simulink subsystem "PvtSubSys_LATC"  (R2020b)
settings: Solver=VariableStepAuto  StartTime=0.0  StopTime=10.0  RelTol=1e-3
values from neighbouring files (symbols this model uses):
  P_Global_CharSpd_ms : value not decoded    [PubParsGlobal.sldd]
  P_Global_SteeringAngleRatio : value not decoded    [PubParsGlobal.sldd]
  P_Global_WheelBase_m : value not decoded    [PubParsGlobal.sldd]
  P_LCS_A0_Limit = 0.25    [LATC.sldd]    (also in LCS_v05.sldd)
  P_LCS_A1_Limit = 0.002    [LATC.sldd]    (also in LCS_v05.sldd)
  P_LCS_communicationTest = 1.0    [LATC.sldd]    (also in LCS_v05.sldd)
  P_LCS_Current_Offset_Test_SW = 0.0    [LATC.sldd]
  P_LCS_Current_Offset_Test_Value = 0.0    [LATC.sldd]
  P_LCS_Curvature_bp : value not decoded    [LATC.sldd]
  P_LCS_CycleTime = 0.4 0.4 0.4 0.4 0.4 0.4 0.4 0.4 0.4 0.6 0.6 0.6 0.6 0.6 0.6 0.6 0.4 0.4 0.4 0.4 0.4 0.4 0.4 0.4 0.4 0.6 0.6 0.6 0.6 0.6 0.6 0.6 0.4 0.4 0.4 0.4 0.4 0.4 0.4 0.4 0.4 0.6 0.6 0.6 0.6 0.6 0.6 0.6 0.4 0.4 0.4 0.4 0.4 0.4 0.4 0.4 0.4 0.6 0.6 0.6 0.6 0.6 0.6 0.6 0.4 0.4 0.4 0.4 0.4 0.4 0.4 0.4 0.4 0.6 0.6 0.6 0.6 0.6 0.6 0.6 0.4 0.4 0.4 0.4 0.4 0.4 0.4 0.4 0.4 0.6 0.6 0.6 0.6 0.6 0.6 0.6 0.4 0.4 0.4 0.4    [LATC.sldd]
  P_LCS_ESS_AngleSlope_Limit = 2.9    [LATC.sldd]    (also in LCS_v05.sldd)
  P_LCS_IN_Offset_Test_SW = 0.0    [LATC.sldd]    (also in LCS_v05.sldd)
  P_LCS_IN_Offset_Test_Value = 0.0    [LATC.sldd]    (also in LCS_v05.sldd)
  P_LCS_LATC_CurOffsetVehicleSpdLimitValue_degs = 7.0    [LATC.sldd]
  P_LCS_LATC_Du_Max = 20.0    [LATC.sldd]
  P_LCS_LATC_ELKAngleSlope_ratio : value not decoded    [LATC.sldd]
  P_LCS_LATC_ELKMaxLatAcc_ms2 : value not decoded    [LATC.sldd]
  P_LCS_LATC_ESSAngleSlope_ratio : value not decoded    [LATC.sldd]
  P_LCS_LATC_ESSMaxLatAcc_ms2 : value not decoded    [LATC.sldd]
  P_LCS_LATC_LCAngleSlope_ratio : value not decoded    [LATC.sldd]
  P_LCS_LATC_LCCancleMaxLatAcc_ms2 : value not decoded    [LATC.sldd]
  P_LCS_LATC_LCEcoAngleSlope_ratio : value not decoded    [LATC.sldd]
  P_LCS_LATC_LCEcoMaxLatAcc_ms2 : value not decoded    [LATC.sldd]
  P_LCS_LATC_LCKAngleSlope_ratio : value not decoded    [LATC.sldd]
  P_LCS_LATC_LCKIEAngleSlope_ratio : value not decoded    [LATC.sldd]
  P_LCS_LATC_LCKIEMaxLatAcc_ms2 : value not decoded    [LATC.sldd]
  P_LCS_LATC_LCKMaxLatAcc_ms2 : value not decoded    [LATC.sldd]
  P_LCS_LATC_LCNormalAngleSlope_ratio : value not decoded    [LATC.sldd]
  P_LCS_LATC_LCNormalMaxLatAcc_ms2 : value not decoded    [LATC.sldd]
  P_LCS_LATC_LCSportAngleSlope_ratio : value not decoded    [LATC.sldd]
  P_LCS_LATC_LCSportMaxLatAcc_ms2 : value not decoded    [LATC.sldd]
  P_LCS_LATC_LKAAngleSlope_ratio : value not decoded    [LATC.sldd]
  P_LCS_LATC_LKAMaxLatAcc_ms2 : value not decoded    [LATC.sldd]
  P_LCS_LATC_MatrixQ1_st = 0.8 0.8 1.2 1.4 1.4 1.4 2.0 2.2 2.2 2.2 2.2 2.2 2.2 2.2 2.2 2.2 0.8 0.8 1.2 1.4 1.4 1.4 2.0 2.2 2.2 2.2 2.2 2.2 2.2 2.2 2.2 2.2 0.8 0.8 1.2 1.4 1.4 1.4 2.0 2.2 2.2 2.2 2.2 2.2 2.2 2.2 2.2 2.2 0.8 0.8 1.2 1.4 1.4 1.4 2.0 2.2 2.2 2.2 2.2 2.2 2.2 2.2 2.2 2.2 0.8 0.8 1.2 1.4 1.4 1.4 2.0 2.2 2.2 2.2 2.2 2.2 2.2 2.2 2.2 2.2 0.8 0.8 1.2 1.4 1.4 1.4 2.0 2.2 2.2 2.2 2.2 2.2 2.2 2.2 2.2 2.2 0.8 0.8 1.2 1.4    [LATC.sldd]
  P_LCS_LATC_MatrixQ3_st = 20.0 20.0 20.0 20.0 20.0 15.0 15.0 15.0 15.0 15.0 15.0 15.0 15.0 13.0 13.0 13.0 20.0 20.0 20.0 20.0 20.0 15.0 15.0 15.0 15.0 15.0 15.0 15.0 15.0 13.0 13.0 13.0 20.0 20.0 20.0 20.0 20.0 15.0 15.0 15.0 15.0 15.0 15.0 15.0 15.0 13.0 13.0 13.0 20.0 20.0 20.0 20.0 20.0 15.0 15.0 15.0 15.0 15.0 15.0 15.0 15.0 13.0 13.0 13.0 20.0 20.0 20.0 20.0 20.0 15.0 15.0 15.0 15.0 15.0 15.0 15.0 15.0 13.0 13.0 13.0    [LATC.sldd]
  P_LCS_LATC_MatrixR_st = 10.0 10.0 10.0 10.0 10.0 10.0 10.0 15.0 15.0 15.0 15.0 15.0 15.0 15.0 15.0 15.0 10.0 10.0 10.0 10.0 10.0 10.0 10.0 15.0 15.0 15.0 15.0 15.0 15.0 15.0 15.0 15.0 10.0 10.0 10.0 10.0 10.0 10.0 10.0 15.0 15.0 15.0 15.0 15.0 15.0 15.0 15.0 15.0 10.0 10.0 10.0 10.0 10.0 10.0 10.0 15.0 15.0 15.0 15.0 15.0 15.0 15.0 15.0 15.0 10.0 10.0 10.0 10.0 10.0 10.0 10.0 15.0 15.0 15.0 15.0 15.0 15.0 15.0 15.0 15.0    [LATC.sldd]
  P_LCS_LATC_Max_LatAcc = 4.0    [LATC.sldd]
  P_LCS_LATC_Max_Phi = 15.0    [LATC.sldd]
  P_LCS_LATC_Max_y = 0.5    [LATC.sldd]
  P_LCS_LATC_MPC_SW = 0.0    [LATC.sldd]
  P_LCS_LATC_PreView_SW = 1.0    [LATC.sldd]
  P_LCS_LATC_SoftConstWeight = 1.0    [LATC.sldd]
  P_LCS_LATC_StateActivAngleSlopeLimit_ratio : value not decoded    [LATC.sldd]
  P_LCS_LATC_StateActiveFlg_TabX_st : value not decoded    [LATC.sldd]
  P_LCS_LATC_StateActiveHoldTime_TabY_st : value not decoded    [LATC.sldd]
  P_LCS_LATC_StateHoldTime_st = 250.0    [LATC.sldd]
  P_LCS_LATC_TarAngleFliterWindowSize = 5.0    [LATC.sldd]
  P_LCS_LATC_TarAngleLP_Time = 0.02    [LATC.sldd]
  P_LCS_LATC_U_Max = 90.0    [LATC.sldd]
  P_LCS_LCK_AngleSlope_Limit = 1.4    [LATC.sldd]
  P_LCS_LineVaildSW = 0.0    [LATC.sldd]
  P_LCS_Lookahead_Distance : value not decoded    [LATC.sldd]
  P_LCS_Lookahead_DistanceFac : value not decoded    [LATC.sldd]
  P_LCS_PLAN_CurvePreView_s = 0.3    [LATC.sldd]
  P_LCS_PLAN_CurvePreview_TabX_m : value not decoded    [LATC.sldd]
  P_LCS_PLAN_CurvePreViewFilterTime_s = 0.1    [LATC.sldd]
  P_LCS_PLAN_ELKAyDtLimit_Tab_ms3 = 1.0 1.0 1.0 1.0 1.0 1.0 1.0 1.0 1.0 1.0 1.0 1.0 1.0 1.0 1.0 1.0 1.0 1.0 1.0 1.0 1.0 1.0 1.0 1.0 1.0 1.0 1.0 1.0 1.0 1.0 1.0 1.0 1.0 1.0 1.0 1.0 1.0 1.0 1.0 1.0 1.0 1.0 1.0 1.0 1.0 1.0 1.0 1.0 1.0 1.0 1.0 1.0 1.0 1.0 1.0 1.0 1.0 1.0 1.0 1.0 1.0 1.0 1.0 1.0 1.0 1.0 1.0 1.0 1.0 1.0 1.0 1.0 1.0 1.0 1.0 1.0 1.0 1.0 1.0 1.0 1.0 1.0 1.0 1.0 1.0 1.0 1.0 1.0 1.0 1.0 1.0 1.0 1.0 1.0 1.0 1.0 1.0 1.0 1.0 1.0    [LATC.sldd]
  P_LCS_PLAN_ESSAyDtLimit_Tab_ms3 = 1.0 1.0 1.0 1.0 1.0 1.0 1.0 1.0 1.0 1.0 1.0 1.0 1.0 1.0 1.0 1.0 1.0 1.0 1.0 1.0 1.0 1.0 1.0 1.0 1.0 1.0 1.0 1.0 1.0 1.0 1.0 1.0 1.0 1.0 1.0 1.0 1.0 1.0 1.0 1.0 1.0 1.0 1.0 1.0 1.0 1.0 1.0 1.0 1.0 1.0 1.0 1.0 1.0 1.0 1.0 1.0 1.0 1.0 1.0 1.0 1.0 1.0 1.0 1.0 1.0 1.0 1.0 1.0 1.0 1.0 1.0 1.0 1.0 1.0 1.0 1.0 1.0 1.0 1.0 1.0 1.0 1.0 1.0 1.0 1.0 1.0 1.0 1.0 1.0 1.0 1.0 1.0 1.0 1.0 1.0 1.0 1.0 1.0 1.0 1.0    [LATC.sldd]
  P_LCS_PLAN_LCCancleAyDtLimit_Tab_ms3 = 1.0 1.0 1.0 1.0 1.0 1.0 1.0 1.0 1.0 1.0 1.0 1.0 1.0 1.0 1.0 1.0 1.0 1.0 1.0 1.0 1.0 1.0 1.0 1.0 1.0 1.0 1.0 1.0 1.0 1.0 1.0 1.0 1.0 1.0 1.0 1.0 1.0 1.0 1.0 1.0 1.0 1.0 1.0 1.0 1.0 1.0 1.0 1.0 1.0 1.0 1.0 1.0 1.0 1.0 1.0 1.0 1.0 1.0 1.0 1.0 1.0 1.0 1.0 1.0 1.0 1.0 1.0 1.0 1.0 1.0 1.0 1.0 1.0 1.0 1.0 1.0 1.0 1.0 1.0 1.0 1.0 1.0 1.0 1.0 1.0 1.0 1.0 1.0 1.0 1.0 1.0 1.0 1.0 1.0 1.0 1.0 1.0 1.0 1.0 1.0    [LATC.sldd]
  P_LCS_PLAN_LCEcoAyDtLimit_Tab_ms3 = 1.0 1.0 1.0 1.0 1.0 1.0 1.0 1.0 1.0 1.0 1.0 1.0 1.0 1.0 1.0 1.0 1.0 1.0 1.0 1.0 1.0 1.0 1.0 1.0 1.0 1.0 1.0 1.0 1.0 1.0 1.0 1.0 1.0 1.0 1.0 1.0 1.0 1.0 1.0 1.0 1.0 1.0 1.0 1.0 1.0 1.0 1.0 1.0 1.0 1.0 1.0 1.0 1.0 1.0 1.0 1.0 1.0 1.0 1.0 1.0 1.0 1.0 1.0 1.0 1.0 1.0 1.0 1.0 1.0 1.0 1.0 1.0 1.0 1.0 1.0 1.0 1.0 1.0 1.0 1.0 1.0 1.0 1.0 1.0 1.0 1.0 1.0 1.0 1.0 1.0 1.0 1.0 1.0 1.0 1.0 1.0 1.0 1.0 1.0 1.0    [LATC.sldd]
  P_LCS_PLAN_LCKAyDtLimit_Tab_ms3 = 1.5 1.5 1.5 1.5 1.5 1.5 1.5 1.5 1.5 1.5 1.5 1.5 1.5 1.5 1.5 1.5 1.5 1.5 1.5 1.5 1.5 1.5 1.5 1.5 1.5 1.5 1.5 1.5 1.5 1.5 1.5 1.5 1.5 1.5 1.5 1.5 1.5 1.5 1.5 1.5 1.5 1.5 1.5 1.5 1.5 1.5 1.5 1.5 1.5 1.5 1.5 1.5 1.5 1.5 1.5 1.5 1.5 1.5 1.5 1.5 1.5 1.5 1.5 1.5 1.5 1.5 1.5 1.5 1.5 1.5 1.5 1.5 1.5 1.5 1.5 1.5 1.5 1.5 1.5 1.5 1.5 1.5 1.5 1.5 1.5 1.5 1.5 1.5 1.5 1.5 1.5 1.5 1.5 1.5 1.5 1.5 1.5 1.5 1.5 1.5    [LATC.sldd]
  P_LCS_PLAN_LCKIEAyDtLimit_Tab_ms3 = 1.0 1.0 1.0 1.0 1.0 1.0 1.0 1.0 1.0 1.0 1.0 1.0 1.0 1.0 1.0 1.0 1.0 1.0 1.0 1.0 1.0 1.0 1.0 1.0 1.0 1.0 1.0 1.0 1.0 1.0 1.0 1.0 1.0 1.0 1.0 1.0 1.0 1.0 1.0 1.0 1.0 1.0 1.0 1.0 1.0 1.0 1.0 1.0 1.0 1.0 1.0 1.0 1.0 1.0 1.0 1.0 1.0 1.0 1.0 1.0 1.0 1.0 1.0 1.0 1.0 1.0 1.0 1.0 1.0 1.0 1.0 1.0 1.0 1.0 1.0 1.0 1.0 1.0 1.0 1.0 1.0 1.0 1.0 1.0 1.0 1.0 1.0 1.0 1.0 1.0 1.0 1.0 1.0 1.0 1.0 1.0 1.0 1.0 1.0 1.0    [LATC.sldd]
  P_LCS_PLAN_LCNormalAyDtLimit_Tab_ms3 = 1.0 1.0 1.0 1.0 1.0 1.0 1.0 1.0 1.0 1.0 1.0 1.0 1.0 1.0 1.0 1.0 1.0 1.0 1.0 1.0 1.0 1.0 1.0 1.0 1.0 1.0 1.0 1.0 1.0 1.0 1.0 1.0 1.0 1.0 1.0 1.0 1.0 1.0 1.0 1.0 1.0 1.0 1.0 1.0 1.0 1.0 1.0 1.0 1.0 1.0 1.0 1.0 1.0 1.0 1.0 1.0 1.0 1.0 1.0 1.0 1.0 1.0 1.0 1.0 1.0 1.0 1.0 1.0 1.0 1.0 1.0 1.0 1.0 1.0 1.0 1.0 1.0 1.0 1.0 1.0 1.0 1.0 1.0 1.0 1.0 1.0 1.0 1.0 1.0 1.0 1.0 1.0 1.0 1.0 1.0 1.0 1.0 1.0 1.0 1.0    [LATC.sldd]
  P_LCS_PLAN_LCSportAyDtLimit_Tab_ms3 = 1.0 1.0 1.0 1.0 1.0 1.0 1.0 1.0 1.0 1.0 1.0 1.0 1.0 1.0 1.0 1.0 1.0 1.0 1.0 1.0 1.0 1.0 1.0 1.0 1.0 1.0 1.0 1.0 1.0 1.0 1.0 1.0 1.0 1.0 1.0 1.0 1.0 1.0 1.0 1.0 1.0 1.0 1.0 1.0 1.0 1.0 1.0 1.0 1.0 1.0 1.0 1.0 1.0 1.0 1.0 1.0 1.0 1.0 1.0 1.0 1.0 1.0 1.0 1.0 1.0 1.0 1.0 1.0 1.0 1.0 1.0 1.0 1.0 1.0 1.0 1.0 1.0 1.0 1.0 1.0 1.0 1.0 1.0 1.0 1.0 1.0 1.0 1.0 1.0 1.0 1.0 1.0 1.0 1.0 1.0 1.0 1.0 1.0 1.0 1.0    [LATC.sldd]
  P_LCS_PLAN_LKAAyDtLimit_Tab_ms3 = 1.0 1.0 1.0 1.0 1.0 1.0 1.0 1.0 1.0 1.0 1.0 1.0 1.0 1.0 1.0 1.0 1.0 1.0 1.0 1.0 1.0 1.0 1.0 1.0 1.0 1.0 1.0 1.0 1.0 1.0 1.0 1.0 1.0 1.0 1.0 1.0 1.0 1.0 1.0 1.0 1.0 1.0 1.0 1.0 1.0 1.0 1.0 1.0 1.0 1.0 1.0 1.0 1.0 1.0 1.0 1.0 1.0 1.0 1.0 1.0 1.0 1.0 1.0 1.0 1.0 1.0 1.0 1.0 1.0 1.0 1.0 1.0 1.0 1.0 1.0 1.0 1.0 1.0 1.0 1.0 1.0 1.0 1.0 1.0 1.0 1.0 1.0 1.0 1.0 1.0 1.0 1.0 1.0 1.0 1.0 1.0 1.0 1.0 1.0 1.0    [LATC.sldd]
  P_LCS_PLAN_MinPlanDis_m : value not decoded    [LATC.sldd]
  P_LCS_PLAN_PreCurMinDisFac_ratio : value not decoded    [LATC.sldd]
  P_LCS_PLAN_PreDisCurve_TabX_m : value not decoded    [LATC.sldd]
  P_LCS_PLAN_StateActiv_AyDtLimit_ms3 : value not decoded    [LATC.sldd]
  P_LCS_PLAN_VehicleSpd_TabX_kph : value not decoded    [LATC.sldd]
  P_LCS_PLAN_VehicleSpd_TabY_Kph : value not decoded    [LATC.sldd]
  P_LCS_Trq_Switch = 0.0    [LATC.sldd]    (also in LCS_v05.sldd)
  P_LCS_VehicleSpd_TabX_Kph : value not decoded    [LATC.sldd]
undefined symbols (not defined in the file or in its folder): HWP_AngCmdReqVal, HWP_AngCmdReqValVld, HWP_FuncTrqCmdReqFlag, HWP_ReqCtrlEPS, HWP_ReqCtrlEPSVld, HWP_TrqOvlCmdReqValue, HWP_WorkReq, HWP_WorkReqVld
libraries: simulink x4, dspbuff3 x2
(part 3 of 8)

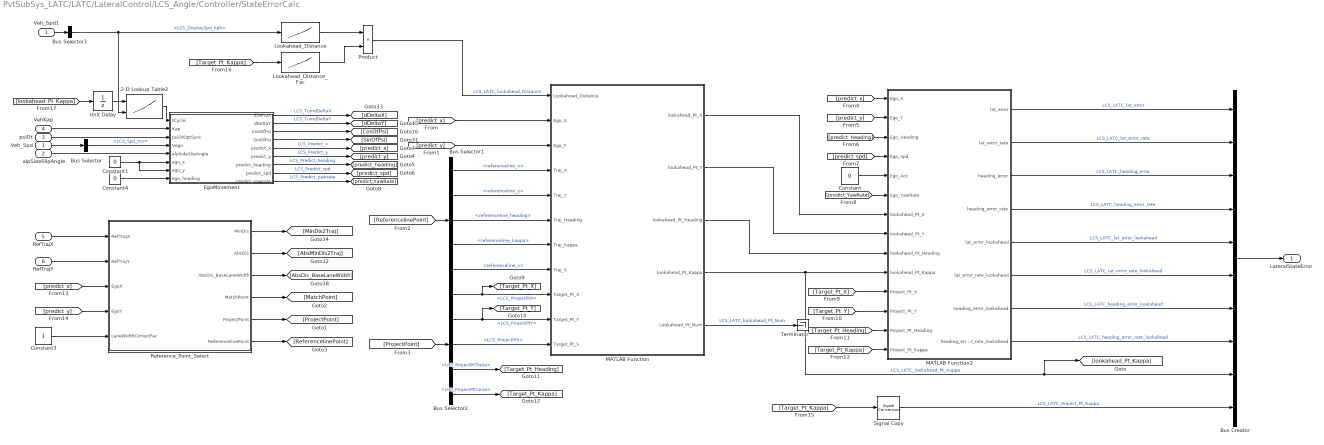
== system PvtSubSys_LATC/LATC/LateralControl/LCS_Angle/Controller/StateErrorCalc ==
  Veh_Spd : Inport
  alpSideSlipAngle : Inport  Port=2
  psiDt : Inport  Port=3
  VehKap : Inport  Port=4
  RefTrajX : Inport  Port=5
  RefTrajY : Inport  Port=6
  2-D Lookup Table2 : Lookup_n-D  BreakpointsForDimension1=P_LCS_Curvature_bp  BreakpointsForDimension2=P_LCS_VehicleSpd_TabX_Kph  Table=P_LCS_CycleTime  InternalRulePriority=Speed  RndMeth=Simplest  InputSameDT=on
      settings: InputPortMap=u0,u1
  Bus Creator : BusCreator  Inputs=10
  Bus Selector : BusSelector  OutputSignals=LCS_Spd_ms
  Bus Selector1 : BusSelector  OutputSignals=referenceline_x,referenceline_y,referenceline_heading,referenceline_kappa,referenceline_s
  Bus Selector2 : BusSelector  OutputSignals=LCS_ProjectPtX,LCS_ProjectPtY,LCS_ProjectPtS,LCS_ProjectPtTheta,LCS_ProjectPtCurve
  Bus Selector3 : BusSelector  OutputSignals=LCS_DisplaySpd_kph
  Constant : Constant  Value=0  OutDataTypeStr=single
  Constant1 : Constant  Value=0  OutDataTypeStr=single
  Constant3 : Constant  OutDataTypeStr=single
  Constant4 : Constant  Value=0  OutDataTypeStr=single
  EgoMovement : MATLAB Function  TreatAsAtomicUnit=on
  Lookahead_Distance : Lookup_n-D  NumberOfTableDimensions=1  BreakpointsForDimension1=P_LCS_VehicleSpd_TabX_Kph  Table=P_LCS_Lookahead_Distance  ExtrapMethod=Clip  UseLastTableValue=on  InternalRulePriority=Speed  RndMeth=Simplest  InputSameDT=on
  Lookahead_Distance_Fac : Lookup_n-D  NumberOfTableDimensions=1  BreakpointsForDimension1=P_LCS_Curvature_bp  Table=P_LCS_Lookahead_DistanceFac  ExtrapMethod=Clip  UseLastTableValue=on  InternalRulePriority=Speed  RndMeth=Simplest  InputSameDT=on
  MATLAB Function : MATLAB Function  TreatAsAtomicUnit=on
  MATLAB Function2 : MATLAB Function  TreatAsAtomicUnit=on
  Product : Product
  Reference_Point_Select : Subsystem
  Signal Copy : SignalConversion  OverrideOpt=off
  Terminator : Terminator
  Unit Delay : UnitDelay  SampleTime=-1  HasFrameUpgradeWarning=on
  Veh_Spd1 : InportShadow
  LateralStateError : Outport
  wires:
  Unit Delay/1 -> 2-D Lookup Table2/1
  Veh_Spd1/1 -> Bus Selector3/1
  [lookahead_Pt_Kappa] -> Unit Delay/1
  2-D Lookup Table2/1 -> EgoMovement/1(tCycle)
  Lookahead_Distance_Fac/1 -> Product/2
  Lookahead_Distance/1 -> Product/1
  [Target_Pt_Kappa] -> Lookahead_Distance_Fac/1
  Bus Selector3/1 -> Lookahead_Distance/1, 2-D Lookup Table2/2  "<LCS_DisplaySpd_kph>"
  [Target_Pt_Kappa] -> Signal Copy/1
  Constant/1 -> MATLAB Function2/5(Ego_Acc)
  MATLAB Function/2(lookahead_Pt_Y) -> MATLAB Function2/8(lookahead_Pt_Y)
  [predict_YawRate] -> MATLAB Function2/6(Ego_YawRate)
  [Target_Pt_Heading] -> MATLAB Function2/13(Project_Pt_Heading)
  MATLAB Function/1(lookahead_Pt_X) -> MATLAB Function2/7(lookahead_Pt_X)
  MATLAB Function/4(lookahead_Pt_Kappa) -> MATLAB Function2/10(lookahead_Pt_Kappa), [lookahead_Pt_Kappa], Bus Creator/9  "LCS_LATC_lookahead_Pt_Kappa"
  MATLAB Function2/1(lat_error) -> Bus Creator/1  "LCS_LATC_lat_error"
  MATLAB Function/5(Lookahead_Pt_Num) -> Terminator/1  "LCS_LATC_lookahead_Pt_Num"
  [Target_Pt_X] -> MATLAB Function2/11(Project_Pt_X)
  [Target_Pt_Kappa] -> MATLAB Function2/14(Project_Pt_Kappa)
  [predict_heading] -> MATLAB Function2/3(Ego_Heading)
  MATLAB Function2/4(heading_error_rate) -> Bus Creator/4  "LCS_LATC_heading_error_rate"
  MATLAB Function2/2(lat_error_rate) -> Bus Creator/2  "LCS_LATC_lat_error_rate"
  [predict_y] -> MATLAB Function2/2(Ego_Y)
  MATLAB Function2/3(heading_error) -> Bus Creator/3  "LCS_LATC_heading_error"
  [Target_Pt_Y] -> MATLAB Function2/12(Project_Pt_Y)
  Bus Creator/1 -> LateralStateError/1
  MATLAB Function/3(lookahead_Pt_Heading) -> MATLAB Function2/9(lookahead_Pt_Heading)
  [predict_x] -> MATLAB Function2/1(Ego_X)
  [predict_spd] -> MATLAB Function2/4(Ego_Spd)
  MATLAB Function2/6(lat_error_rate_lookahead) -> Bus Creator/6  "LCS_LATC_lat_error_rate_lookahead"
  MATLAB Function2/8(heading_error_rate_lookahead) -> Bus Creator/8  "LCS_LATC_heading_error_rate_lookahead"
  MATLAB Function2/7(heading_error_lookahead) -> Bus Creator/7  "LCS_LATC_heading_error_lookahead"
  MATLAB Function2/5(lat_error_lookahead) -> Bus Creator/5  "LCS_LATC_lat_error_lookahead"
  Signal Copy/1 -> Bus Creator/10  "LCS_LATC_Project_Pt_Kappa"
  [predict_y] -> Reference_Point_Select/4(EgoY)
  [predict_x] -> Reference_Point_Select/3(EgoX)
  Product/1 -> MATLAB Function/1(Lookahead_Distance)  "LCS_LATC_lookahead_Distance"
  Constant4/1 -> EgoMovement/8(ego_heading)
  Constant1/1 -> EgoMovement/6(ego_x), EgoMovement/7(ego_y)
  Bus Selector2/5 -> [Target_Pt_Kappa]  "<LCS_ProjectPtCurve>"
  Bus Selector2/4 -> [Target_Pt_Heading]  "<LCS_ProjectPtTheta>"
  Bus Selector2/3 -> MATLAB Function/11(Target_Pt_S)  "<LCS_ProjectPtS>"
  Bus Selector2/1 -> [Target_Pt_X], MATLAB Function/9(Target_Pt_X)  "<LCS_ProjectPtX>"
  Bus Selector2/2 -> [Target_Pt_Y], MATLAB Function/10(Target_Pt_Y)  "<LCS_ProjectPtY>"
  [ProjectPoint] -> Bus Selector2/1
  Bus Selector1/5 -> MATLAB Function/8(Traj_S)  "<referenceline_s>"
  Bus Selector1/4 -> MATLAB Function/7(Traj_Kappa)  "<referenceline_kappa>"
  Bus Selector1/3 -> MATLAB Function/6(Traj_Heading)  "<referenceline_heading>"
  Bus Selector1/2 -> MATLAB Function/5(Traj_Y)  "<referenceline_y>"
  Bus Selector1/1 -> MATLAB Function/4(Traj_X)  "<referenceline_x>"
  [ReferencelinePoint] -> Bus Selector1/1
  [predict_y] -> MATLAB Function/3(Ego_Y)
  [predict_x] -> MATLAB Function/2(Ego_X)
  EgoMovement/9(predict_yawrate) -> [predict_YawRate]  "LCS_Predict_yawrate"
  EgoMovement/8(predict_spd) -> [predict_spd]  "LCS_Predict_spd"
  EgoMovement/7(predict_heading) -> [predict_heading]  "LCS_Predict_heading"
  EgoMovement/6(predict_y) -> [predict_y]  "LCS_Predict_y"
  EgoMovement/5(predict_x) -> [predict_x]  "LCS_Predict_x"
  Reference_Point_Select/6(ReferencelinePoint) -> [ReferencelinePoint]
  Reference_Point_Select/5(ProjectPoint) -> [ProjectPoint]
  Reference_Point_Select/4(MatchPoint) -> [MatchPoint]
  RefTrajY/1 -> Reference_Point_Select/2(RefTrajY)
  Constant3/1 -> Reference_Point_Select/5(LaneWidthCorrectFac)
  RefTrajX/1 -> Reference_Point_Select/1(RefTrajX)
  Reference_Point_Select/1(MinDis) -> [MinDis2Traj]
  Reference_Point_Select/2(AbsDis) -> [AbsMinDis2Traj]
  Reference_Point_Select/3(AbsDis_BaseLaneWidth) -> [AbsDis_BaseLaneWidth]
  EgoMovement/2(dDeltaY) -> [dDeltaY]  "LCS_TurndDeltaY"
  psiDt/1 -> EgoMovement/3(psiDtOptSync)
  alpSideSlipAngle/1 -> EgoMovement/5(alpSideSlipAngle)
  Veh_Spd/1 -> Bus Selector/1
  EgoMovement/3(CosOfPsi) -> [CosOfPsi]
  VehKap/1 -> EgoMovement/2(Kap)
  EgoMovement/4(SinOfPsi) -> [SinOfPsi]
  EgoMovement/1(dDeltaX) -> [dDeltaX]  "LCS_TurndDeltaX"
  Bus Selector/1 -> EgoMovement/4(Vego)  "<LCS_Spd_ms>"

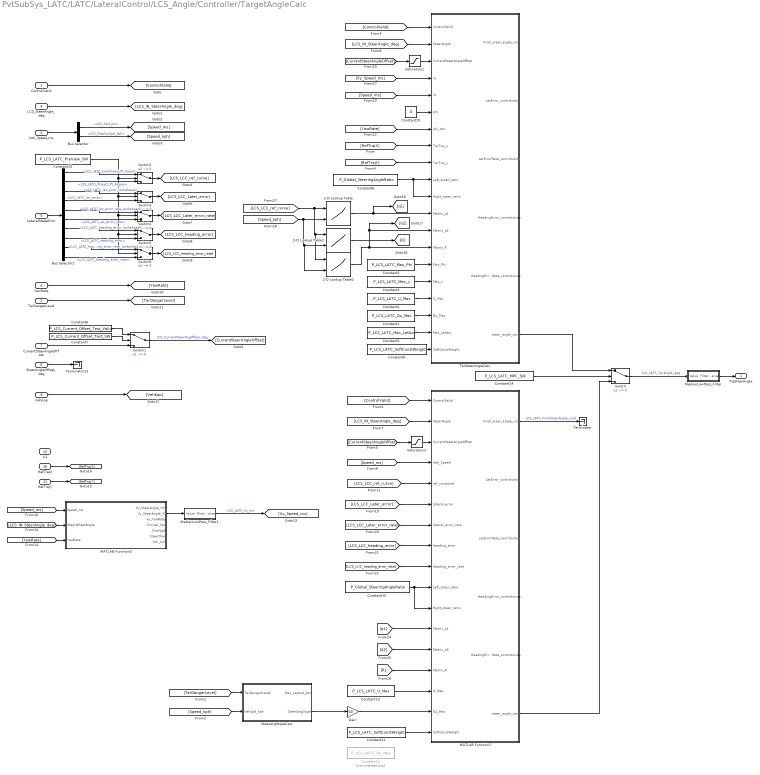
== system PvtSubSys_LATC/LATC/LateralControl/LCS_Angle/Controller/TargetAngleCalc ==
  ControlValid : Inport
  TarDangerLevel : Inport  Port=2
  Veh_Speed_ms : Inport  Port=3
  LCS_SteerAngle_deg : Inport  Port=4
  LateralStateError : Inport  Port=5
  YawRate : Inport  Port=6
  CurrentSteerAngleOffset : Inport  Port=7
  SteerAngleOffset_deg : Inport  Port=8
  VehKap : Inport  Port=9
  RefTrajX : Inport  Port=10
  RefTrajY : Inport  Port=11
  A1 : Inport  Port=12
  2-D Lookup Table : Lookup_n-D  BreakpointsForDimension1=P_LCS_Curvature_bp  BreakpointsForDimension2=P_LCS_VehicleSpd_TabX_Kph  Table=P_LCS_LATC_MatrixQ1_st  InternalRulePriority=Speed  RndMeth=Simplest  InputSameDT=on
      settings: InputPortMap=u0,u1
  2-D Lookup Table1 : Lookup_n-D  BreakpointsForDimension1=P_LCS_Curvature_bp  BreakpointsForDimension2=P_LCS_VehicleSpd_TabX_Kph  Table=P_LCS_LATC_MatrixQ3_st  InternalRulePriority=Speed  RndMeth=Simplest  InputSameDT=on
      settings: InputPortMap=u0,u1
  2-D Lookup Table2 : Lookup_n-D  BreakpointsForDimension1=P_LCS_Curvature_bp  BreakpointsForDimension2=P_LCS_VehicleSpd_TabX_Kph  Table=P_LCS_LATC_MatrixR_st  InternalRulePriority=Speed  RndMeth=Simplest  InputSameDT=on
      settings: InputPortMap=u0,u1
  Bus Selector : BusSelector  OutputSignals=LCS_Spd_ms,LCS_DisplaySpd_kph
  Bus Selector1 : BusSelector  OutputSignals=LCS_LATC_lookahead_Pt_Kappa,LCS_LATC_Project_Pt_Kappa,LCS_LATC_lat_error_lookahead,LCS_LATC_lat_error,LCS_LATC_lat_error_rate_lookahead,LCS_LATC_lat_error_rate,LCS_LATC_heading_error_lookahead,LCS_LATC_heading_error,LCS_LATC_heading_error_rate_lookahead,LCS_LATC_heading_error_rate
  Constant1 : Constant  Value=P_LCS_LATC_Du_Max  OutDataTypeStr=single
  Constant10 : Constant  Value=P_Global_SteeringAngleRatio  OutDataTypeStr=single
  Constant11 : Constant  Value=P_LCS_LATC_SoftConstWeight  OutDataTypeStr=single
  Constant12 : Constant  Commented=on  Value=P_LCS_LATC_Du_Max  OutDataTypeStr=single
  Constant13 : Constant  Value=P_LCS_LATC_U_Max  OutDataTypeStr=single
  Constant14 : Constant  Value=P_LCS_LATC_MPC_SW  OutDataTypeStr=single
  Constant15 : Constant  Value=P_LCS_LATC_PreView_SW  OutDataTypeStr=single
  Constant19 : Constant  Value=0  OutDataTypeStr=single
  Constant2 : Constant  Value=P_LCS_LATC_Max_Phi  OutDataTypeStr=single
  Constant3 : Constant  Value=P_LCS_LATC_Max_y  OutDataTypeStr=single
  Constant4 : Constant  Value=P_LCS_LATC_U_Max  OutDataTypeStr=single
  Constant5 : Constant  Value=P_LCS_LATC_Max_LatAcc  OutDataTypeStr=single
  Constant6 : Constant  Value=P_Global_SteeringAngleRatio  OutDataTypeStr=single
  Constant7 : Constant  Description=0  Value=P_LCS_Current_Offset_Test_SW  OutDataTypeStr=uint8
      settings: AttributesFormatString=%<Description>
  Constant8 : Constant  Description=0  Value=P_LCS_Current_Offset_Test_Value  OutDataTypeStr=single
      settings: AttributesFormatString=%<Description>
  Constant9 : Constant  Value=P_LCS_LATC_SoftConstWeight  OutDataTypeStr=single
  Gain : Gain  Gain=50
  MATLAB Function1 : MATLAB Function  TreatAsAtomicUnit=on
  MATLAB Function3 : MATLAB Function  TreatAsAtomicUnit=on
  MedianLowPass_Filter : Subsystem
  MedianLowPass_Filter1 : Subsystem
  Saturation1 : Saturate  UpperLimit=8  LowerLimit=-8  OutDataTypeStr=single
  Saturation2 : Saturate  UpperLimit=8  LowerLimit=-8  OutDataTypeStr=single
  SteerAngSlopeCalc : Subsystem
  Switch{,1..6} (7 alike) : Switch  Criteria=u2 ~= 0
  TarSteerAngleCalc : MATLAB Function  TreatAsAtomicUnit=on
  Terminator : Terminator
  Terminator13 : Terminator
  TrgSteerAngle : Outport  OutDataTypeStr=single
  wires:
  [YawRate] -> MATLAB Function3/3(YawRate)
  [LCS_IN_SteerAngle_deg] -> MATLAB Function3/2(SteerWheelAngle)
  MATLAB Function3/2(Vy_SteerAngle_Kv) -> MedianLowPass_Filter1/1(Value)
  Gain/1 -> MATLAB Function1/16(Du_Max)
  SteerAngSlopeCalc/2(SteerAngSlope) -> Gain/1
  MATLAB Function1/1(Final_steer_angle_cmd) -> Terminator/1  "LCS_LATC_FinalSteerAngle_cmd"
  [Speed_kph] -> 2-D Lookup Table/2, 2-D Lookup Table1/2, 2-D Lookup Table2/2
  [LCS_LCC_ref_curve] -> 2-D Lookup Table/1, 2-D Lookup Table1/1, 2-D Lookup Table2/1
  Constant15/1 -> Switch2/2, Switch3/2, Switch4/2, Switch5/2, Switch6/2
  Bus Selector1/9 -> Switch6/1  "<LCS_LATC_heading_error_rate_lookahead>"
  Bus Selector1/10 -> Switch6/3  "<LCS_LATC_heading_error_rate>"
  Switch6/1 -> [LCS_LCC_heading_error_rate]
  Bus Selector1/7 -> Switch5/1  "<LCS_LATC_heading_error_lookahead>"
  Bus Selector1/8 -> Switch5/3  "<LCS_LATC_heading_error>"
  Switch5/1 -> [LCS_LCC_heading_error]
  Bus Selector1/5 -> Switch4/1  "<LCS_LATC_lat_error_rate_lookahead>"
  Bus Selector1/6 -> Switch4/3  "<LCS_LATC_lat_error_rate>"
  Switch4/1 -> [LCS_LCC_Later_error_rate]
  Bus Selector1/4 -> Switch3/3  "<LCS_LATC_lat_error>"
  Bus Selector1/3 -> Switch3/1  "<LCS_LATC_lat_error_lookahead>"
  Switch3/1 -> [LCS_LCC_Later_error]
  Bus Selector1/2 -> Switch2/3  "<LCS_LATC_Project_Pt_Kappa>"
  Bus Selector1/1 -> Switch2/1  "<LCS_LATC_lookahead_Pt_Kappa>"
  Switch2/1 -> [LCS_LCC_ref_curve]
  Constant14/1 -> Switch/2
  MATLAB Function1/6(steer_angle_cmd) -> Switch/3
  TarSteerAngleCalc/6(steer_angle_cmd) -> Switch/1
  [R] -> MATLAB Function1/14(Matrix_R)
  [q2] -> MATLAB Function1/13(Matrix_q3)
  [q1] -> MATLAB Function1/12(Matrix_q1)
  Constant13/1 -> MATLAB Function1/15(U_Max)
  MedianLowPass_Filter/1(FilterValue) -> TrgSteerAngle/1
  Switch/1 -> MedianLowPass_Filter/1(Value)  "LCS_LATC_TarAngle_deg"
  Constant11/1 -> MATLAB Function1/17(SoftConstWeight)
  Constant10/1 -> MATLAB Function1/10(Left_steer_ratio), MATLAB Function1/11(Right_steer_ratio)
  [LCS_LCC_heading_error] -> MATLAB Function1/8(heading_error)
  [LCS_LCC_heading_error_rate] -> MATLAB Function1/9(heading_error_rate)
  [LCS_LCC_Later_error_rate] -> MATLAB Function1/7(lateral_error_rate)
  [LCS_LCC_Later_error] -> MATLAB Function1/6(lateral_error)
  [LCS_LCC_ref_curve] -> MATLAB Function1/5(ref_curvature)
  [Speed_ms] -> MATLAB Function1/4(Veh_Speed)
  [ControlValid] -> MATLAB Function1/1(ControlValid)
  [LCS_IN_SteerAngle_deg] -> MATLAB Function1/2(SteerAngle)
  [CurrentSteerAngleOffset] -> Saturation2/1
  Saturation2/1 -> MATLAB Function1/3(CurrentSteerAngleOffset)
  Constant9/1 -> TarSteerAngleCalc/20(SoftConstWeight)
  Switch1/1 -> [CurrentSteerAngleOffset]  "LCS_CurrentSteerAngOffset_deg"
  CurrentSteerAngleOffset/1 -> Switch1/3
  Constant8/1 -> Switch1/1
  Constant7/1 -> Switch1/2
  Constant5/1 -> TarSteerAngleCalc/19(Max_LatAcc)
  Constant1/1 -> TarSteerAngleCalc/18(Du_Max)
  [RefTrajY] -> TarSteerAngleCalc/9(TarTraj_y)
  [RefTrajX] -> TarSteerAngleCalc/8(TarTraj_x)
  RefTrajY/1 -> [RefTrajY]
  RefTrajX/1 -> [RefTrajX]
  Constant4/1 -> TarSteerAngleCalc/17(U_Max)
  Constant3/1 -> TarSteerAngleCalc/16(Max_y)
  Constant2/1 -> TarSteerAngleCalc/15(Max_Phi)
  2-D Lookup Table1/1 -> TarSteerAngleCalc/13(Matrix_q2), [q2]
  2-D Lookup Table2/1 -> TarSteerAngleCalc/14(Matrix_R), [R]
  2-D Lookup Table/1 -> TarSteerAngleCalc/12(Matrix_q1), [q1]
  [Vy_Speed_ms] -> TarSteerAngleCalc/4(vy)
  MedianLowPass_Filter1/1(FilterValue) -> [Vy_Speed_ms]  "LCS_LATC_Vy_ms"
  [Speed_ms] -> MATLAB Function3/1(Speed_ms)
  Saturation1/1 -> TarSteerAngleCalc/3(CurrentSteerAngleOffset)
  [CurrentSteerAngleOffset] -> Saturation1/1
  VehKap/1 -> [VehKap]
  Constant6/1 -> TarSteerAngleCalc/10(Left_steer_ratio), TarSteerAngleCalc/11(Right_steer_ratio)
  [YawRate] -> TarSteerAngleCalc/7(phi_dot)
  Constant19/1 -> TarSteerAngleCalc/6(phi)
  [Speed_ms] -> TarSteerAngleCalc/5(vx)
  [LCS_IN_SteerAngle_deg] -> TarSteerAngleCalc/2(SteerAngle)
  [ControlValid] -> TarSteerAngleCalc/1(ControlValid)
  LateralStateError/1 -> Bus Selector1/1
  Bus Selector/2 -> [Speed_kph]  "<LCS_DisplaySpd_kph>"
  Bus Selector/1 -> [Speed_ms]  "<LCS_Spd_ms>"
  Veh_Speed_ms/1 -> Bus Selector/1
  YawRate/1 -> [YawRate]
  TarDangerLevel/1 -> [TarDangerLevel]
  ControlValid/1 -> [ControlValid]
  SteerAngleOffset_deg/1 -> Terminator13/1
  LCS_SteerAngle_deg/1 -> [LCS_IN_SteerAngle_deg]
  [TarDangerLevel] -> SteerAngSlopeCalc/1(TarDangerlLevel)
  [Speed_kph] -> SteerAngSlopeCalc/2(VehSpd_kph)

== system PvtSubSys_LATC/LATC/LateralControl/LCS_Angle/Controller/Understeer&Offset_Calc ==
  note: %% 匀速
  SteerAngle_deg : Inport
  PsiDtOpt : Inport  Port=2
  axvRef : Inport  Port=3
  Veh_Spd : Inport  Port=4
  Abs2 : Abs
  Bus Selector : BusSelector  OutputSignals=LCS_Spd_ms
  Compare To Constant1 : simulink/Logic and Bit Operations/Compare To Constant  relop=>  const=P_LCS_LATC_CurOffsetVehicleSpdLimitValue_degs  OutDataTypeStr=boolean
  Compare To Constant6 : simulink/Logic and Bit Operations/Compare To Constant  relop=<=  const=1.5  OutDataTypeStr=boolean
  Constant1 : Constant  Value=P_Global_SteeringAngleRatio
  Constant4 : Constant  Value=P_Global_CharSpd_ms
  Constant5 : Constant  Value=P_Global_WheelBase_m
  Constant6 : Constant  Value=57.3  OutDataTypeStr=single
  Enabled Subsystem : Subsystem  TreatAsAtomicUnit=on
  FilterTime2 : Product  Inputs=*//  RndMeth=Zero
  Logical Operator : Logic  AllPortsSameDT=off  OutDataTypeStr=boolean
  Memory52 : Memory  InheritSampleTime=on
  Sum : Sum  Inputs=+-
  Terminator : Terminator
  YOD_Ackman : MATLAB Function  TreatAsAtomicUnit=on
  SteerAngleOffset_deg : Outport
  wires:
  Veh_Spd/1 -> Bus Selector/1
  Compare To Constant6/1 -> Logical Operator/1
  Abs2/1 -> Compare To Constant6/1
  axvRef/1 -> Abs2/1
  FilterTime2/1 -> YOD_Ackman/4(AlpWheelAngle)
  YOD_Ackman/1(AckConst) -> Enabled Subsystem/1(AckConst)
  Constant6/1 -> FilterTime2/3
  Constant1/1 -> FilterTime2/2
  Logical Operator/1 -> Terminator/1, Enabled Subsystem/Enable  "LCS_OffSetUpdate_Flg"
  Sum/1 -> Enabled Subsystem/2(Raw)
  Bus Selector/1 -> Compare To Constant1/1, YOD_Ackman/1(VxvRef)  "<LCS_Spd_ms>"
  PsiDtOpt/1 -> Sum/2
  Memory52/1 -> YOD_Ackman/5(PsiDtAckK1)
  Constant4/1 -> YOD_Ackman/2(Vch)
  Constant5/1 -> YOD_Ackman/3(WheelBase)
  Enabled Subsystem/1(SteerAngleOffset_deg) -> SteerAngleOffset_deg/1  "LCS_LATC_CurrentSteerAngleOffset_deg"
  YOD_Ackman/2(PsiDtAck) -> Sum/1, Memory52/1
  Compare To Constant1/1 -> Logical Operator/2
  SteerAngle_deg/1 -> FilterTime2/1

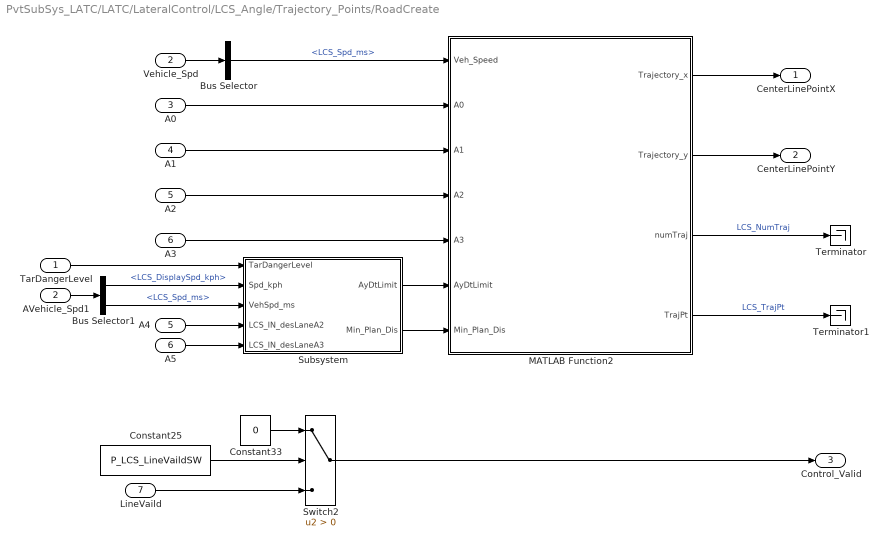
== system PvtSubSys_LATC/LATC/LateralControl/LCS_Angle/Trajectory_Points/RoadCreate ==
  TarDangerLevel : Inport
  Vehicle_Spd : Inport  Port=2  OutDataTypeStr=single
  A0 : Inport  Port=3  OutDataTypeStr=single
  A1 : Inport  Port=4
  A2 : Inport  Port=5
  A3 : Inport  Port=6
  LineVaild : Inport  Port=7
  A4 : InportShadow  Port=5
  A5 : InportShadow  Port=6
  AVehicle_Spd1 : InportShadow  Port=2  OutDataTypeStr=single
  Bus Selector : BusSelector  OutputSignals=LCS_Spd_ms
  Bus Selector1 : BusSelector  OutputSignals=LCS_DisplaySpd_kph,LCS_Spd_ms
  Constant25 : Constant  Value=P_LCS_LineVaildSW
  Constant33 : Constant  Value=0  OutDataTypeStr=boolean
  MATLAB Function2 : MATLAB Function  TreatAsAtomicUnit=on
  Subsystem : Subsystem
  Switch2 : Switch  Criteria=u2 > Threshold
  Terminator : Terminator
  Terminator1 : Terminator
  CenterLinePointX : Outport
  CenterLinePointY : Outport  Port=2
  Control_Valid : Outport  Port=3  OutDataTypeStr=boolean
  wires:
  MATLAB Function2/4(TrajPt) -> Terminator1/1  "LCS_TrajPt"
  MATLAB Function2/3(numTraj) -> Terminator/1  "LCS_NumTraj"
  A5/1 -> Subsystem/5(LCS_IN_desLaneA3)
  A4/1 -> Subsystem/4(LCS_IN_desLaneA2)
  TarDangerLevel/1 -> Subsystem/1(TarDangerLevel)
  Bus Selector1/2 -> Subsystem/3(VehSpd_ms)  "<LCS_Spd_ms>"
  Bus Selector1/1 -> Subsystem/2(Spd_kph)  "<LCS_DisplaySpd_kph>"
  AVehicle_Spd1/1 -> Bus Selector1/1
  Bus Selector/1 -> MATLAB Function2/1(Veh_Speed)  "<LCS_Spd_ms>"
  Vehicle_Spd/1 -> Bus Selector/1
  Subsystem/2(Min_Plan_Dis) -> MATLAB Function2/7(Min_Plan_Dis)
  Subsystem/1(AyDtLimit) -> MATLAB Function2/6(AyDtLimit)
  MATLAB Function2/2(Trajectory_y) -> CenterLinePointY/1
  MATLAB Function2/1(Trajectory_x) -> CenterLinePointX/1
  A3/1 -> MATLAB Function2/5(A3)
  A2/1 -> MATLAB Function2/4(A2)
  A1/1 -> MATLAB Function2/3(A1)
  A0/1 -> MATLAB Function2/2(A0)
  Constant25/1 -> Switch2/2
  LineVaild/1 -> Switch2/3
  Constant33/1 -> Switch2/1
  Switch2/1 -> Control_Valid/1
